simulink model "wah"  (R2014a)
settings: Solver=ode45  StartTime=0.0  StopTime=10.0  RelTol=1e-3
libraries: dspsigops x4, dspsrcs4 x1, dspsnks4 x1
settings Model: Creator=Besims  LastModifiedBy=Besims

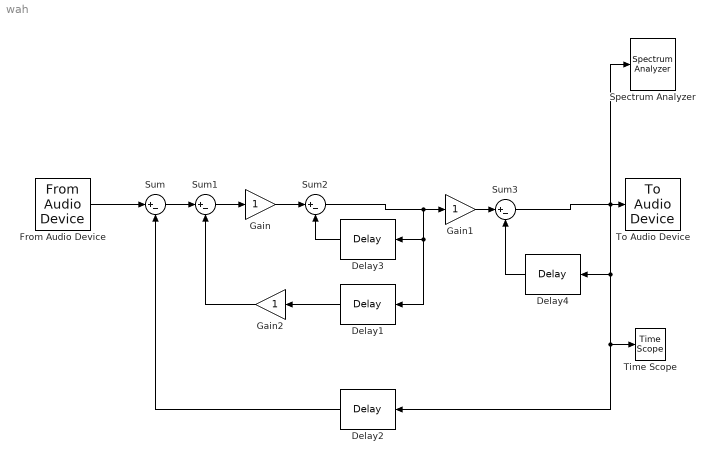
== system wah ==
  Delay{1..4} (4 alike) : dspsigops/Delay  InputProcessing=Columns as channels (frame based)  dly_unit=Samples  delay=1  ic_detail=off  dif_ic_for_ch=off  dif_ic_for_dly=off  ic=0  reset_popup=None
  From Audio Device : dspsrcs4/From Audio Device  deviceName=Mikrofon Dizisi (Realtek High Definition Audio)  numChannels=2  sampleRate=44100  deviceDatatype=Determine from output data type  autoBufferSize=on  bufferSize=4096  queueDuration=1.0  frameSize=1024  outputDatatype=double  defaultInputChannelMapping=on  inputChannelMapping=1:2
  Gain : Gain
  Gain1 : Gain
  Gain2 : Gain
  Spectrum Analyzer : SpectrumAnalyzer
  Sum{,1..3} (4 alike) : Sum  Inputs=|+-
  Time Scope : TimeScope  DefaultConfigurationName=spbscopes.TimeScopeBlockCfg
  To Audio Device : dspsnks4/To Audio Device  deviceName=Hoparlör/Kulaklık (Realtek High Definition Audio)  inheritSampleRate=on  sampleRate=44100  deviceDatatype=Determine from input data type  autoBufferSize=on  bufferSize=4096  queueDuration=1.0  defaultOutputChannelMapping=on  outputChannelMapping=1:2
  wires:
  From Audio Device/1 -> Sum/1
  Sum/1 -> Sum1/1
  Delay2/1 -> Sum/2
  Sum1/1 -> Gain/1
  Gain/1 -> Sum2/1
  Delay3/1 -> Sum2/2
  Sum2/1 -> Delay3/1, Delay1/1, Gain1/1
  Delay4/1 -> Sum3/2
  Gain1/1 -> Sum3/1
  Sum3/1 -> Spectrum Analyzer/1, Time Scope/1, Delay2/1, Delay4/1, To Audio Device/1
  Delay1/1 -> Gain2/1
  Gain2/1 -> Sum1/2
